simulink model "controller_design"  (R2014b)
settings: Solver=ode45  StartTime=0.0  StopTime=10.0  RelTol=1e-3
libraries: simulink x1
settings Model: Creator=Ugo Pattacini  LastModifiedBy=Ugo Pattacini

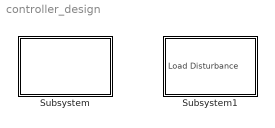
== system controller_design ==
  Subsystem : Subsystem
  Subsystem1 : Subsystem

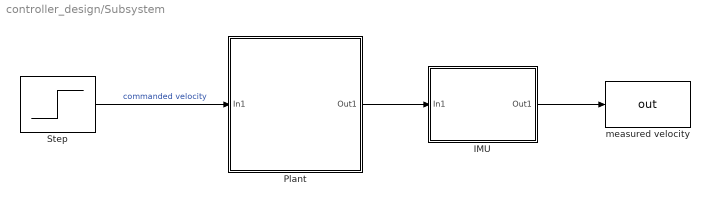
== system controller_design/Subsystem ==
  IMU : Subsystem
      mask Display: image('imu.jpg')
  Plant : Subsystem
      mask Display: image('icub-head.png')
  Step : Step  SampleTime=0
  measured velocity : ToWorkspace  VariableName=out  SaveFormat=Timeseries  SampleTime=-1
  wires:
  Plant/1(Out1) -> IMU/1(In1)
  Step/1 -> Plant/1(In1)  "commanded velocity"
  IMU/1(Out1) -> measured velocity/1

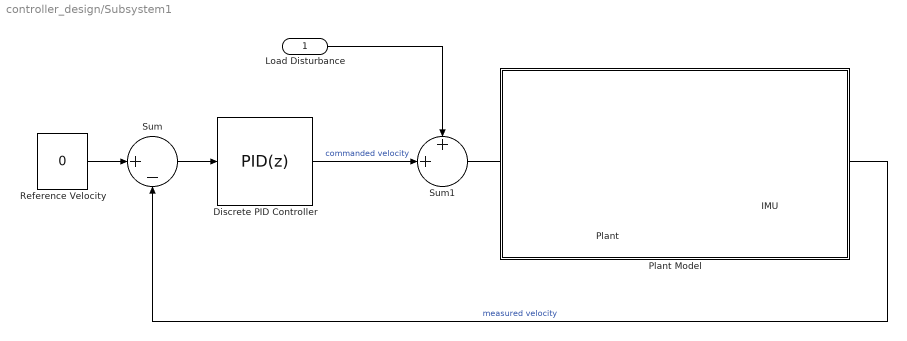
== system controller_design/Subsystem1 ==
  Load Disturbance : Inport
  Discrete PID Controller : simulink/Continuous/PID Controller  Controller=PID  TimeDomain=Discrete-time  SampleTime=1  IntegratorMethod=Forward Euler  FilterMethod=Forward Euler  Form=Parallel  P=1  I=1  D=0  N=100  InitialConditionSource=internal  InitialConditionForIntegrator=0  InitialConditionForFilter=0  ExternalReset=none  LimitOutput=off  UpperSaturationLimit=inf  LowerSaturationLimit=-inf  LinearizeAsGain=off  AntiWindupMode=none  Kb=1  TrackingMode=off  Kt=1  PParamMin=[]  PParamMax=[]  IParamMin=[]  IParamMax=[]  DParamMin=[]  DParamMax=[]  NParamMin=[]  NParamMax=[]  KbParamMin=[]  KbParamMax=[]  KtParamMin=[]  KtParamMax=[]  POutMin=[]  POutMax=[]  IOutMin=[]  IOutMax=[]  DOutMin=[]  DOutMax=[]  NOutMin=[]  NOutMax=[]  KbOutMin=[]  KbOutMax=[]  KtOutMin=[]  KtOutMax=[]  IntegratorOutMin=[]  IntegratorOutMax=[]  FilterOutMin=[]  FilterOutMax=[]  SumOutMin=[]  SumOutMax=[]  SumI1OutMin=[]  SumI1OutMax=[]  SumI2OutMin=[]  SumI2OutMax=[]  SumI3OutMin=[]  SumI3OutMax=[]  SumDOutMin=[]  SumDOutMax=[]  SaturationOutMin=[]  SaturationOutMax=[]  IntegratorContinuousStateAttributes=''  IntegratorStateMustResolveToSignalObject=off  IntegratorRTWStateStorageClass=Auto  FilterContinuousStateAttributes=''  FilterStateMustResolveToSignalObject=off  FilterRTWStateStorageClass=Auto  DifferentiatorICPrevScaledInput=0  DifferentiatorOutMin=[]  DifferentiatorOutMax=[]  UseFilter=on
  IMU : Subsystem
      mask Display: image('imu.jpg')
  Plant : Subsystem
      mask Display: image('icub-head.png')
  Plant Model : Subsystem
  Reference Velocity : Constant  Value=0
  Sum : Sum  Inputs=|+-
  Sum1 : Sum  Inputs=++|
  wires:
  Sum1/1 -> Plant/1(In1)
  IMU/1(Out1) -> Sum/2  "measured velocity"
  Reference Velocity/1 -> Sum/1
  Discrete PID Controller/1 -> Sum1/2  "commanded velocity"
  Load Disturbance/1 -> Sum1/1
  Sum/1 -> Discrete PID Controller/1
  Plant/1(Out1) -> IMU/1(In1)

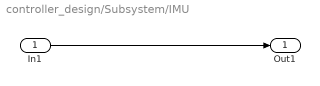
== system controller_design/Subsystem/IMU ==
  In1 : Inport
  Out1 : Outport
  wires:
  In1/1 -> Out1/1

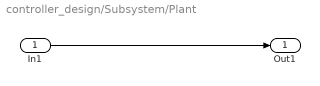
== system controller_design/Subsystem/Plant ==
  In1 : Inport
  Out1 : Outport
  wires:
  In1/1 -> Out1/1

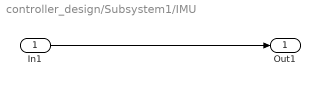
== system controller_design/Subsystem1/IMU ==
  In1 : Inport
  Out1 : Outport
  wires:
  In1/1 -> Out1/1

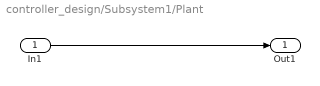
== system controller_design/Subsystem1/Plant ==
  In1 : Inport
  Out1 : Outport
  wires:
  In1/1 -> Out1/1

== system controller_design/Subsystem1/Plant Model ==
